simulink model "FlightDataRecorder"  (R2023b)
settings: Solver=VariableStepAuto  StartTime=0.0  StopTime=inf  RelTol=1e-3
libraries: dspindex x28, simulink x4, dspnetwork x4, etargetslib x3, aerolibconvert2 x1
(part 2 of 3)

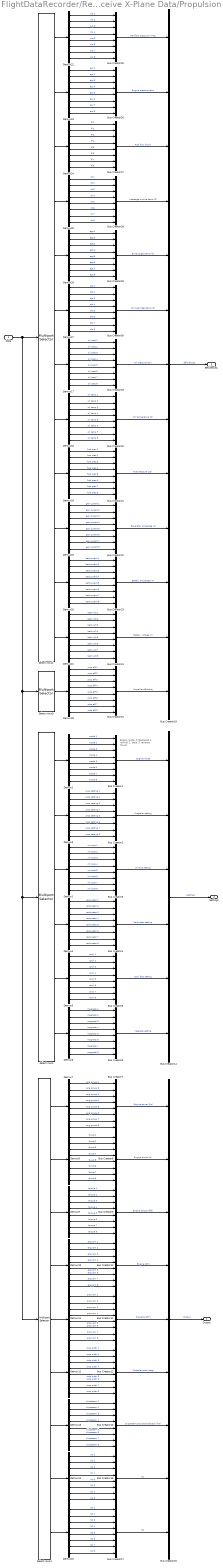
== system FlightDataRecorder/Receive X-Plane Data/Propulsion data ==
  note: Engine mode:
      | 0: feathered
      | 1: normal
      | 2: 'beta'
      | 3: reverse thrust
  Data : Inport
  Bus Creator{1..13,16..18,20..31} (28 alike) : BusCreator  Inputs=8
  Bus Creator14 : BusCreator  Inputs=6
  Bus Creator15 : BusCreator  Inputs=9
  Bus Creator19 : BusCreator  Inputs=13
  Demux{1..28} (28 alike) : Demux  Outputs=8
  Select rows : dspindex/Multiport Selector  rowsOrCols=Rows  idxCellArray={28,29,30,31,32,33}  idxErrMode=Clip Index
  Select rows1 : dspindex/Multiport Selector  rowsOrCols=Rows  idxCellArray={35,36,37,38,39,40,41,42,43}  idxErrMode=Clip Index
  Select rows2 : dspindex/Multiport Selector  rowsOrCols=Rows  idxCellArray={44,45,46,47,48,49,50,51,52,53,54,55}  idxErrMode=Clip Index
  Select rows3 : dspindex/Multiport Selector  rowsOrCols=Rows  idxCellArray={70}  idxErrMode=Clip Index
  Output : Outport
  Settings : Outport  Port=2
  Efficiencies : Outport  Port=3
  wires:
  Demux3/3 -> Bus Creator2/3  "prop setting 3"
  Demux3/2 -> Bus Creator2/2  "prop setting 2"
  Demux3/1 -> Bus Creator2/1  "prop setting 1"
  Demux3/4 -> Bus Creator2/4  "prop setting 4"
  Demux3/5 -> Bus Creator2/5  "prop setting 5"
  Demux3/6 -> Bus Creator2/6  "prop setting 6"
  Demux3/7 -> Bus Creator2/7  "prop setting 7"
  Demux3/8 -> Bus Creator2/8  "prop setting 8"
  Select rows/1 -> Demux2/1
  Select rows/2 -> Demux3/1
  Demux2/8 -> Bus Creator1/8  "mode 8"
  Demux2/1 -> Bus Creator1/1  "mode 1"
  Demux2/4 -> Bus Creator1/4  "mode 4"
  Demux2/7 -> Bus Creator1/7  "mode 7"
  Demux2/3 -> Bus Creator1/3  "mode 3"
  Demux2/5 -> Bus Creator1/5  "mode 5"
  Demux2/6 -> Bus Creator1/6  "mode 6"
  Demux2/2 -> Bus Creator1/2  "mode 2"
  Bus Creator1/1 -> Bus Creator14/1  "Engine mode"
  Bus Creator2/1 -> Bus Creator14/2  "Propeller setting"
  Demux1/3 -> Bus Creator3/3  "mixture 3"
  Demux1/4 -> Bus Creator3/4  "mixture 4"
  Demux1/5 -> Bus Creator3/5  "mixture 5"
  Demux1/6 -> Bus Creator3/6  "mixture 6"
  Demux1/7 -> Bus Creator3/7  "mixture 7"
  Demux1/8 -> Bus Creator3/8  "mixture 8"
  Select rows/3 -> Demux1/1
  Bus Creator3/1 -> Bus Creator14/3  "Mixture setting"
  Demux1/1 -> Bus Creator3/1  "mixture 1"
  Demux1/2 -> Bus Creator3/2  "mixture 2"
  Select rows/4 -> Demux4/1
  Demux4/4 -> Bus Creator4/4  "carburetor 4"
  Demux4/1 -> Bus Creator4/1  "carburetor 1"
  Demux4/6 -> Bus Creator4/6  "carburetor 6"
  Demux4/7 -> Bus Creator4/7  "carburetor 7"
  Demux4/5 -> Bus Creator4/5  "carburetor 5"
  Demux4/3 -> Bus Creator4/3  "carburetor 3"
  Demux4/2 -> Bus Creator4/2  "carburetor 2"
  Demux4/8 -> Bus Creator4/8  "carburetor 8"
  Bus Creator4/1 -> Bus Creator14/4  "Carburetor setting"
  Demux5/4 -> Bus Creator5/4  "cowl 4"
  Demux5/1 -> Bus Creator5/1  "cowl 1"
  Demux5/6 -> Bus Creator5/6  "cowl 6"
  Demux5/7 -> Bus Creator5/7  "cowl 7"
  Demux5/5 -> Bus Creator5/5  "cowl 5"
  Demux5/3 -> Bus Creator5/3  "cowl 3"
  Demux5/2 -> Bus Creator5/2  "cowl 2"
  Demux5/8 -> Bus Creator5/8  "cowl 8"
  Bus Creator5/1 -> Bus Creator14/5  "Cowl flap setting"
  Select rows/5 -> Demux5/1
  Demux6/4 -> Bus Creator6/4  "magneto 4"
  Demux6/1 -> Bus Creator6/1  "magneto 1"
  Demux6/6 -> Bus Creator6/6  "magneto 6"
  Demux6/7 -> Bus Creator6/7  "magneto 7"
  Demux6/5 -> Bus Creator6/5  "magneto 5"
  Demux6/3 -> Bus Creator6/3  "magneto 3"
  Demux6/2 -> Bus Creator6/2  "magneto 2"
  Demux6/8 -> Bus Creator6/8  "magneto 8"
  Bus Creator6/1 -> Bus Creator14/6  "Magneto setting"
  Select rows/6 -> Demux6/1
  Demux7/4 -> Bus Creator7/4  "eng power 4"
  Demux7/1 -> Bus Creator7/1  "eng power 1"
  Demux7/6 -> Bus Creator7/6  "eng power 6"
  Demux7/7 -> Bus Creator7/7  "eng power 7"
  Demux7/5 -> Bus Creator7/5  "eng power 5"
  Demux7/3 -> Bus Creator7/3  "eng power 3"
  Demux7/2 -> Bus Creator7/2  "eng power 2"
  Demux7/8 -> Bus Creator7/8  "eng power 8"
  Select rows1/1 -> Demux7/1
  Demux8/4 -> Bus Creator8/4  "thrust 4"
  Demux8/1 -> Bus Creator8/1  "thrust 1"
  Demux8/6 -> Bus Creator8/6  "thrust 6"
  Demux8/7 -> Bus Creator8/7  "thrust 7"
  Demux8/5 -> Bus Creator8/5  "thrust 5"
  Demux8/3 -> Bus Creator8/3  "thrust 3"
  Demux8/2 -> Bus Creator8/2  "thrust 2"
  Demux8/8 -> Bus Creator8/8  "thrust 8"
  Select rows1/2 -> Demux8/1
  Demux9/4 -> Bus Creator9/4  "torque 4"
  Demux9/1 -> Bus Creator9/1  "torque 1"
  Demux9/6 -> Bus Creator9/6  "torque 6"
  Demux9/7 -> Bus Creator9/7  "torque 7"
  Demux9/5 -> Bus Creator9/5  "torque 5"
  Demux9/3 -> Bus Creator9/3  "torque 3"
  Demux9/2 -> Bus Creator9/2  "torque 2"
  Demux9/8 -> Bus Creator9/8  "torque 8"
  Select rows1/3 -> Demux9/1
  Demux10/4 -> Bus Creator10/4  "eng rpm 4"
  Demux10/1 -> Bus Creator10/1  "eng rpm 1"
  Demux10/6 -> Bus Creator10/6  "eng rpm 6"
  Demux10/7 -> Bus Creator10/7  "eng rpm 7"
  Demux10/5 -> Bus Creator10/5  "eng rpm 5"
  Demux10/3 -> Bus Creator10/3  "eng rpm 3"
  Demux10/2 -> Bus Creator10/2  "eng rpm 2"
  Demux10/8 -> Bus Creator10/8  "eng rpm 8"
  Select rows1/4 -> Demux10/1
  Demux11/4 -> Bus Creator11/4  "prop rpm 4"
  Demux11/1 -> Bus Creator11/1  "prop rpm 1"
  Demux11/6 -> Bus Creator11/6  "prop rpm 6"
  Demux11/7 -> Bus Creator11/7  "prop rpm 7"
  Demux11/5 -> Bus Creator11/5  "prop rpm 5"
  Demux11/3 -> Bus Creator11/3  "prop rpm 3"
  Demux11/2 -> Bus Creator11/2  "prop rpm 2"
  Demux11/8 -> Bus Creator11/8  "prop rpm 8"
  Select rows1/5 -> Demux11/1
  Demux12/4 -> Bus Creator12/4  "prop pitch 4"
  Demux12/1 -> Bus Creator12/1  "prop pitch 1"
  Demux12/6 -> Bus Creator12/6  "prop pitch 6"
  Demux12/7 -> Bus Creator12/7  "prop pitch 7"
  Demux12/5 -> Bus Creator12/5  "prop pitch 5"
  Demux12/3 -> Bus Creator12/3  "prop pitch 3"
  Demux12/2 -> Bus Creator12/2  "prop pitch 2"
  Demux12/8 -> Bus Creator12/8  "prop pitch 8"
  Select rows1/6 -> Demux12/1
  Demux13/4 -> Bus Creator13/4  "slipstream 4"
  Demux13/1 -> Bus Creator13/1  "slipstream 1"
  Demux13/6 -> Bus Creator13/6  "slipstream 6"
  Demux13/7 -> Bus Creator13/7  "slipstream 7"
  Demux13/5 -> Bus Creator13/5  "slipstream 5"
  Demux13/3 -> Bus Creator13/3  "slipstream 3"
  Demux13/2 -> Bus Creator13/2  "slipstream 2"
  Demux13/8 -> Bus Creator13/8  "slipstream 8"
  Select rows1/7 -> Demux13/1
  Bus Creator14/1 -> Settings/1  "Settings"
  Bus Creator7/1 -> Bus Creator15/1  "Engine power (hp)"
  Bus Creator8/1 -> Bus Creator15/2  "Engine thrust (lb)"
  Bus Creator9/1 -> Bus Creator15/3  "Engine torque (ftlb)"
  Bus Creator10/1 -> Bus Creator15/4  "Engine RPM"
  Bus Creator11/1 -> Bus Creator15/5  "Propeller RPM"
  Bus Creator12/1 -> Bus Creator15/6  "Propeller pitch (deg)"
  Bus Creator13/1 -> Bus Creator15/7  "Slipstream/propwash/jetwash (knt)"
  Bus Creator15/1 -> Output/1  "Output"
  Demux14/4 -> Bus Creator16/4  "N1 4"
  Demux14/6 -> Bus Creator16/6  "N1 6"
  Demux14/7 -> Bus Creator16/7  "N1 7"
  Demux14/5 -> Bus Creator16/5  "N1 5"
  Demux14/3 -> Bus Creator16/3  "N1 3"
  Demux14/2 -> Bus Creator16/2  "N1 2"
  Demux14/8 -> Bus Creator16/8  "N1 8"
  Select rows1/8 -> Demux14/1
  Demux15/4 -> Bus Creator17/4  "N2 4"
  Demux15/6 -> Bus Creator17/6  "N2 6"
  Demux15/7 -> Bus Creator17/7  "N2 7"
  Demux15/5 -> Bus Creator17/5  "N2 5"
  Demux15/3 -> Bus Creator17/3  "N2 3"
  Demux15/2 -> Bus Creator17/2  "N2 2"
  Demux15/8 -> Bus Creator17/8  "N2 8"
  Select rows1/9 -> Demux15/1
  Demux14/1 -> Bus Creator16/1  "N1 1"
  Demux15/1 -> Bus Creator17/1  "N2 1"
  Bus Creator16/1 -> Bus Creator15/8  "N1"
  Bus Creator17/1 -> Bus Creator15/9  "N2"
  Demux18/3 -> Bus Creator20/3  "oil temp 3"
  Demux18/2 -> Bus Creator20/2  "oil temp 2"
  Demux18/1 -> Bus Creator20/1  "oil temp 1"
  Data/1 -> Select rows3/1, Select rows/1, Select rows1/1, Select rows2/1
  Demux18/4 -> Bus Creator20/4  "oil temp 4"
  Demux18/5 -> Bus Creator20/5  "oil temp 5"
  Demux18/6 -> Bus Creator20/6  "oil temp 6"
  Demux18/7 -> Bus Creator20/7  "oil temp 7"
  Demux18/8 -> Bus Creator20/8  "oil temp 8"
  Demux17/8 -> Bus Creator18/8  "oil pres 8"
  Demux17/1 -> Bus Creator18/1  "oil pres 1"
  Demux17/4 -> Bus Creator18/4  "oil pres 4"
  Demux17/7 -> Bus Creator18/7  "oil pres 7"
  Demux17/3 -> Bus Creator18/3  "oil pres 3"
  Demux17/5 -> Bus Creator18/5  "oil pres 5"
  Demux17/6 -> Bus Creator18/6  "oil pres 6"
  Demux17/2 -> Bus Creator18/2  "oil pres 2"
  Demux16/3 -> Bus Creator21/3  "fuel pres 3"
  Demux16/4 -> Bus Creator21/4  "fuel pres 4"
  Demux16/5 -> Bus Creator21/5  "fuel pres 5"
  Demux16/6 -> Bus Creator21/6  "fuel pres 6"
  Demux16/7 -> Bus Creator21/7  "fuel pres 7"
  Demux16/8 -> Bus Creator21/8  "fuel pres 8"
  Demux16/1 -> Bus Creator21/1  "fuel pres 1"
  Demux16/2 -> Bus Creator21/2  "fuel pres 2"
  Demux19/4 -> Bus Creator22/4  "gen current 4"
  Demux19/1 -> Bus Creator22/1  "gen current 1"
  Demux19/6 -> Bus Creator22/6  "gen current 6"
  Demux19/7 -> Bus Creator22/7  "gen current 7"
  Demux19/5 -> Bus Creator22/5  "gen current 5"
  Demux19/3 -> Bus Creator22/3  "gen current 3"
  Demux19/2 -> Bus Creator22/2  "gen current 2"
  Demux19/8 -> Bus Creator22/8  "gen current 8"
  Demux20/4 -> Bus Creator23/4  "batt current 4"
  Demux20/1 -> Bus Creator23/1  "batt current 1"
  Demux20/6 -> Bus Creator23/6  "batt current 6"
  Demux20/7 -> Bus Creator23/7  "batt current 7"
  Demux20/5 -> Bus Creator23/5  "batt current 5"
  Demux20/3 -> Bus Creator23/3  "batt current 3"
  Demux20/2 -> Bus Creator23/2  "batt current 2"
  Demux20/8 -> Bus Creator23/8  "batt current 8"
  Demux21/1 -> Bus Creator24/1  "batt volt 1"
  Demux21/2 -> Bus Creator24/2  "batt volt 2"
  Bus Creator19/1 -> Efficiencies/1  "Efficiencies"
  Select rows2/12 -> Demux21/1
  Select rows2/11 -> Demux20/1
  Select rows2/10 -> Demux19/1
  Select rows2/9 -> Demux16/1
  Select rows2/7 -> Demux17/1
  Select rows2/8 -> Demux18/1
  Demux21/7 -> Bus Creator24/7  "batt volt 7"
  Demux21/6 -> Bus Creator24/6  "batt volt 6"
  Demux21/8 -> Bus Creator24/8  "batt volt 8"
  Demux21/3 -> Bus Creator24/3  "batt volt 3"
  Demux21/5 -> Bus Creator24/5  "batt volt 5"
  Demux21/4 -> Bus Creator24/4  "batt volt 4"
  Bus Creator18/1 -> Bus Creator19/7  "Oil pressure (psi)"
  Bus Creator20/1 -> Bus Creator19/8  "Oil temperature (C)"
  Bus Creator21/1 -> Bus Creator19/9  "Fuel pressure (psi)"
  Bus Creator22/1 -> Bus Creator19/10  "Generator amperage (A)"
  Bus Creator23/1 -> Bus Creator19/11  "Battery amperage (A)"
  Bus Creator24/1 -> Bus Creator19/12  "Battery voltage (V)"
  Demux22/8 -> Bus Creator25/8  "mp 8"
  Demux22/1 -> Bus Creator25/1  "mp 1"
  Demux22/4 -> Bus Creator25/4  "mp 4"
  Demux22/7 -> Bus Creator25/7  "mp 7"
  Demux22/3 -> Bus Creator25/3  "mp 3"
  Demux22/5 -> Bus Creator25/5  "mp 5"
  Demux22/6 -> Bus Creator25/6  "mp 6"
  Demux22/2 -> Bus Creator25/2  "mp 2"
  Select rows2/1 -> Demux22/1
  Bus Creator25/1 -> Bus Creator19/1  "Manifold pressure (inHg)"
  Demux23/8 -> Bus Creator26/8  "epr 8"
  Demux23/7 -> Bus Creator26/7  "epr 7"
  Select rows2/2 -> Demux23/1
  Bus Creator26/1 -> Bus Creator19/2  "Engine pressure ratio"
  Demux23/6 -> Bus Creator26/6  "epr 6"
  Demux23/4 -> Bus Creator26/4  "epr 4"
  Demux23/1 -> Bus Creator26/1  "epr 1"
  Demux23/2 -> Bus Creator26/2  "epr 2"
  Demux23/3 -> Bus Creator26/3  "epr 3"
  Demux23/5 -> Bus Creator26/5  "epr 5"
  Demux24/8 -> Bus Creator27/8  "ff 8"
  Demux24/7 -> Bus Creator27/7  "ff 7"
  Demux24/6 -> Bus Creator27/6  "ff 6"
  Demux24/4 -> Bus Creator27/4  "ff 4"
  Demux24/1 -> Bus Creator27/1  "ff 1"
  Demux24/2 -> Bus Creator27/2  "ff 2"
  Demux24/3 -> Bus Creator27/3  "ff 3"
  Demux24/5 -> Bus Creator27/5  "ff 5"
  Select rows2/3 -> Demux24/1
  Bus Creator27/1 -> Bus Creator19/3  "Fuel flow (lb/hr)"
  Demux25/8 -> Bus Creator28/8  "itt 8"
  Demux25/7 -> Bus Creator28/7  "itt 7"
  Demux25/6 -> Bus Creator28/6  "itt 6"
  Demux25/4 -> Bus Creator28/4  "itt 4"
  Demux25/1 -> Bus Creator28/1  "itt 1"
  Demux25/2 -> Bus Creator28/2  "itt 2"
  Demux25/3 -> Bus Creator28/3  "itt 3"
  Demux25/5 -> Bus Creator28/5  "itt 5"
  Select rows2/4 -> Demux25/1
  Bus Creator28/1 -> Bus Creator19/4  "Interstage turbine temp (C)"
  Demux26/8 -> Bus Creator29/8  "egt 8"
  Demux26/7 -> Bus Creator29/7  "egt 7"
  Demux26/6 -> Bus Creator29/6  "egt 6"
  Demux26/4 -> Bus Creator29/4  "egt 4"
  Demux26/2 -> Bus Creator29/2  "egt 2"
  Demux26/3 -> Bus Creator29/3  "egt 3"
  Demux26/5 -> Bus Creator29/5  "egt 5"
  Select rows2/5 -> Demux26/1
  Bus Creator29/1 -> Bus Creator19/5  "Exhaust gas temp (C)"
  Demux27/8 -> Bus Creator30/8  "cht 8"
  Demux27/7 -> Bus Creator30/7  "cht 7"
  Demux27/6 -> Bus Creator30/6  "cht 6"
  Demux27/4 -> Bus Creator30/4  "cht 4"
  Demux27/2 -> Bus Creator30/2  "cht 2"
  Demux27/3 -> Bus Creator30/3  "cht 3"
  Demux27/5 -> Bus Creator30/5  "cht 5"
  Select rows2/6 -> Demux27/1
  Demux27/1 -> Bus Creator30/1  "cht 1"
  Bus Creator30/1 -> Bus Creator19/6  "Cylinder head temp (C)"
  Demux26/1 -> Bus Creator29/1  "egt 1"
  Demux28/8 -> Bus Creator31/8  "prop eff 8"
  Demux28/1 -> Bus Creator31/1  "prop eff 1"
  Demux28/4 -> Bus Creator31/4  "prop eff 4"
  Demux28/7 -> Bus Creator31/7  "prop eff 7"
  Demux28/3 -> Bus Creator31/3  "prop eff 3"
  Demux28/5 -> Bus Creator31/5  "prop eff 5"
  Demux28/6 -> Bus Creator31/6  "prop eff 6"
  Demux28/2 -> Bus Creator31/2  "prop eff 2"
  Select rows3/1 -> Demux28/1
  Bus Creator31/1 -> Bus Creator19/13  "Propeller efficiency"

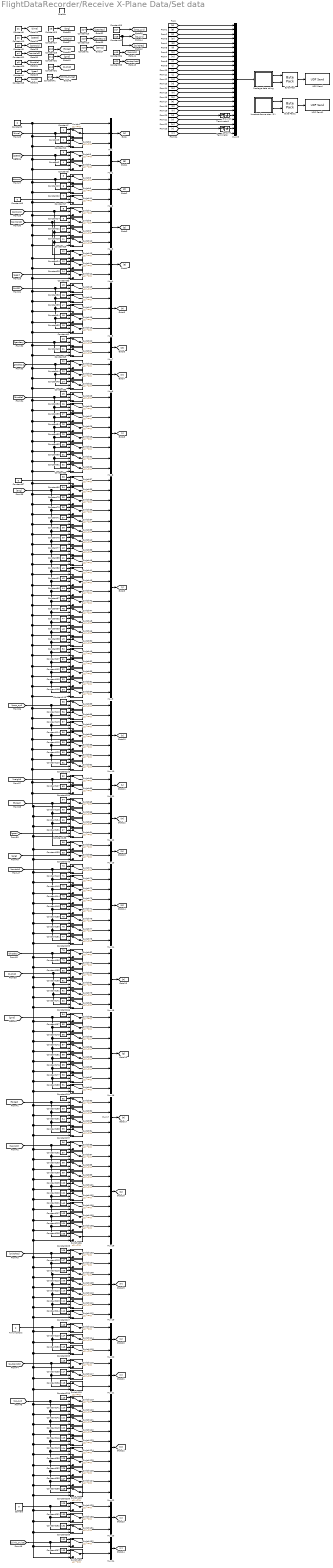
== system FlightDataRecorder/Receive X-Plane Data/Set data ==
  Enable : EnablePort
  Annunciators : Constant  Value=0
  Byte Pack : etargetslib/Byte Pack  datatypes={'uint8','uint32'}  byteAlign=1
  Byte Pack1 : etargetslib/Byte Pack  datatypes={'uint8','uint32'}  byteAlign=1
  Camera : Constant  Value=0
  Constant1 : Constant  Value=p16
  Constant10 : Constant  Value=p2
  Constant102 : Constant  Value=52
  Constant103 : Constant  Value=53
  Constant107 : Constant  Value=51
  Constant108 : Constant  Value=54
  Constant11 : Constant  Value=p4
  Constant110 : Constant  Value=56
  Constant113 : Constant  Value=55
  Constant114 : Constant  Value=58
  Constant115 : Constant  Value=59
  Constant119 : Constant  Value=57
  Constant12 : Constant  Value=3
  Constant120 : Constant  Value=61
  Constant125 : Constant  Value=60
  Constant126 : Constant  Value=62
  Constant127 : Constant  Value=63
  Constant128 : Constant  Value=65
  Constant13 : Constant  Value=6
  Constant131 : Constant  Value=67
  Constant134 : Constant  Value=66
  Constant135 : Constant  Value=64
  Constant138 : Constant  Value=68
  Constant139 : Constant  Value=69
  Constant14 : Constant  Value=9
  Constant140 : Constant  Value=71
  Constant143 : Constant  Value=70
  Constant144 : Constant  Value=73
  Constant145 : Constant  Value=74
  Constant149 : Constant  Value=72
  Constant15 : Constant  Value=p7
  Constant150 : Constant  Value=76
  Constant151 : Constant  Value=77
  Constant155 : Constant  Value=75
  Constant156 : Constant  Value=79
  Constant159 : Constant  Value=78
  Constant16 : Constant  Value=p14
  Constant160 : Constant  Value=81
  Constant161 : Constant  Value=82
  Constant165 : Constant  Value=80
  Constant166 : Constant  Value=84
  Constant167 : Constant  Value=85
  Constant17 : Constant  Value=8
  Constant171 : Constant  Value=83
  Constant172 : Constant  Value=87
  Constant175 : Constant  Value=86
  Constant176 : Constant  Value=89
  Constant177 : Constant  Value=90
  Constant18 : Constant  Value=11
  Constant181 : Constant  Value=88
  Constant183 : Constant  Value=91
  Constant184 : Constant  Value=92
  Constant185 : Constant  Value=93
  Constant188 : Constant  Value=95
  Constant19 : Constant  Value=p15
  Constant191 : Constant  Value=94
  Constant192 : Constant  Value=97
  Constant193 : Constant  Value=98
  Constant197 : Constant  Value=96
  Constant199 : Constant  Value=99
  Constant2 : Constant  Value=4
  Constant20 : Constant  Value=p5
  Constant200 : Constant  Value=101
  Constant201 : Constant  Value=102
  Constant205 : Constant  Value=100
  Constant207 : Constant  Value=103
  Constant208 : Constant  Value=105
  Constant209 : Constant  Value=106
  Constant21 : Constant  Value=10
  Constant213 : Constant  Value=104
  Constant215 : Constant  Value=107
  Constant216 : Constant  Value=108
  Constant219 : Constant  Value=109
  Constant22 : Constant  Value=7
  Constant220 : Constant  Value=110
  Constant223 : Constant  Value=111
  Constant224 : Constant  Value=112
  Constant227 : Constant  Value=113
  Constant229 : Constant  Value=114
  Constant23 : Constant  Value=p8
  Constant230 : Constant  Value=115
  Constant233 : Constant  Value=116
  Constant235 : Constant  Value=117
  Constant236 : Constant  Value=118
  Constant238 : Constant  Value=119
  Constant24 : Constant  Value=13
  Constant241 : Constant  Value=120
  Constant242 : Constant  Value=121
  Constant245 : Constant  Value=122
  Constant246 : Constant  Value=123
  Constant249 : Constant  Value=124
  Constant25 : Constant  Value=14
  Constant250 : Constant  Value=125
  Constant252 : Constant  Value=126
  Constant255 : Constant  Value=127
  Constant256 : Constant  Value=128
  Constant259 : Constant  Value=129
  Constant26 : Constant  Value=p17
  Constant261 : Constant  Value=130
  Constant262 : Constant  Value=131
  Constant265 : Constant  Value=132
  Constant267 : Constant  Value=133
  Constant27 : Constant  Value=p9
  Constant28 : Constant  Value=p10
  Constant29 : Constant  Value=12
  Constant3 : Constant  Value=p3
  Constant30 : Constant  Value=16
  Constant31 : Constant  Value=p12
  Constant32 : Constant  Value=p11
  Constant33 : Constant  Value=15
  Constant34 : Constant  Value=18
  Constant35 : Constant  Value=19
  Constant36 : Constant  Value=p19
  Constant37 : Constant  Value=0
  Constant38 : Constant  Value=p20
  Constant39 : Constant  Value=17
  Constant4 : Constant  Value=p6
  Constant40 : Constant  Value=p18
  Constant41 : Constant  Value=p13
  Constant42 : Constant  Value=20
  Constant43 : Constant  Value=21
  Constant44 : Constant  Value=23
  Constant45 : Constant  Value=24
  Constant46 : Constant  Value=0
  Constant49 : Constant  Value=22
  Constant5 : Constant  Value=0
  Constant50 : Constant  Value=26
  Constant53 : Constant  Value=25
  Constant54 : Constant  Value=28
  Constant55 : Constant  Value=29
  Constant59 : Constant  Value=27
  Constant6 : Constant  Value=5
  Constant60 : Constant  Value=31
  Constant61 : Constant  Value=32
  Constant65 : Constant  Value=30
  Constant66 : Constant  Value=34
  Constant69 : Constant  Value=33
  Constant7 : Constant
  Constant70 : Constant  Value=36
  Constant71 : Constant  Value=37
  Constant75 : Constant  Value=35
  Constant76 : Constant  Value=39
  Constant77 : Constant  Value=40
  Constant8 : Constant  Value=p1
  Constant81 : Constant  Value=38
  Constant82 : Constant  Value=42
  Constant85 : Constant  Value=41
  Constant86 : Constant  Value=44
  Constant87 : Constant  Value=45
  Constant9 : Constant  Value=2
  Constant91 : Constant  Value=43
  Constant92 : Constant  Value=47
  Constant93 : Constant  Value=48
  Constant97 : Constant  Value=46
  Constant98 : Constant  Value=49
  Constant99 : Constant  Value=50
  From : From
  Goto : Goto
  Ground : Ground
  Ground1 : Ground
  Mux{,2,4,6,20..21,23} (7 alike) : Mux  Inputs=3
  Mux{1,7,11,13,24} (5 alike) : Mux  Inputs=2
  Mux10 : Mux  Inputs=7
  Mux12 : Mux
  Mux14 : Mux  Inputs=8
  Mux15 : Mux  Inputs=6
  Mux16 : Mux  Inputs=8
  Mux17 : Mux
  Mux18 : Mux  Inputs=10
  Mux19 : Mux  Inputs=7
  Mux22 : Mux  Inputs=10
  Mux25 : Mux  Inputs=25
  Mux3 : Mux
  Mux5 : Mux  Inputs=5
  Mux8 : Mux  Inputs=8
  Mux9 : Mux  Inputs=22
  Package data string : MATLAB Function  TreatAsAtomicUnit=on
  Switch{1..133} (133 alike) : Switch  Criteria=u2 ~= 0  SaturateOnIntegerOverflow=off  InputSameDT=off
  Terminator : Terminator
  Terminator1 : Terminator
  UDP Send : dspnetwork/UDP Send  remoteURL=ipaddress  remotePort=sport  localURL='0.0.0.0'  localPortSource=Automatically determine  localPort=-1  sendBufferSize=8192  sampletime=-1  blockPlatform=[]  separateLengthPort=0
  UDP Send1 : dspnetwork/UDP Send  remoteURL=ipaddress  remotePort=sport  localURL='0.0.0.0'  localPortSource=Automatically determine  localPort=-1  sendBufferSize=8192  sampletime=-1  blockPlatform=[]  separateLengthPort=0
  Unselect frame rate <0> : MATLAB Function  TreatAsAtomicUnit=on
  wires:
  Constant7/1 -> Switch1/1
  [time] -> Switch2/2, Switch1/2
  Constant9/1 -> Switch2/1
  Constant12/1 -> Switch3/1
  [speed] -> Switch4/2, Switch3/2
  Constant2/1 -> Switch4/1
  Switch1/1 -> Mux/2
  Switch2/1 -> Mux/3
  Switch3/1 -> Mux1/1
  Switch4/1 -> Mux1/2
  Constant6/1 -> Switch5/1
  [atmos] -> Switch6/2, Switch5/2
  Constant13/1 -> Switch6/1
  Constant17/1 -> Switch7/1
  [controls] -> Switch7/2, Switch14/2, Switch10/2, Switch9/2
  Constant14/1 -> Switch8/1
  Constant21/1 -> Switch9/1
  Constant18/1 -> Switch10/1
  Switch7/1 -> Mux3/1
  Switch8/1 -> Mux3/2
  Switch9/1 -> Mux3/3
  Switch10/1 -> Mux3/4
  Switch5/1 -> Mux2/1
  Switch6/1 -> Mux2/2
  Constant22/1 -> Switch11/1
  Switch11/1 -> Mux2/3
  Constant29/1 -> Switch13/1
  Constant24/1 -> Switch14/1
  Switch13/1 -> Mux4/1
  Switch14/1 -> Mux4/2
  Constant25/1 -> Switch12/1
  [gear] -> Switch12/2
  Switch12/1 -> Mux4/3
  Constant33/1 -> Switch19/1
  [AHRS] -> Switch16/2, Switch18/2, Switch17/2, Switch15/2, Switch19/2
  Constant30/1 -> Switch15/1
  Constant39/1 -> Switch17/1
  Constant34/1 -> Switch18/1
  Constant35/1 -> Switch16/1
  Switch18/1 -> Mux5/4
  Switch15/1 -> Mux5/2
  Switch16/1 -> Mux5/5
  Switch17/1 -> Mux5/3
  Switch19/1 -> Mux5/1
  Constant42/1 -> Switch20/1
  [geodesy] -> Switch21/2, Switch20/2
  Constant43/1 -> Switch21/1
  Switch20/1 -> Mux7/1
  Switch21/1 -> Mux7/2
  Constant5/1 -> Mux/1, Switch5/3, Switch11/3, Switch7/3, Switch8/3, Switch9/3, Switch13/3, Switch14/3, Switch12/3, Switch19/3, Switch15/3, Switch17/3, Switch18/3, Switch16/3, Switch20/3, Switch23/3, Switch24/3, Switch22/3, Switch29/3, Switch25/3, Switch27/3, Switch28/3, Switch26/3, Switch31/3, Switch32/3, Switch37/3, Switch33/3, Switch35/3, Switch36/3, Switch34/3, Switch39/3, Switch40/3, Switch38/3, Switch45/3, Switch41/3, Switch43/3, Switch44/3, Switch42/3, Switch47/3, Switch48/3, Switch46/3, Switch50/3, Switch49/3, Switch52/3, Switch53/3, Switch51/3, Switch59/3, Switch55/3, Switch57/3, Switch58/3, Switch56/3, Switch61/3, Switch66/3, Switch67/3, Switch74/3, Switch70/3, Switch72/3, Switch73/3, Switch71/3, Switch76/3, Switch77/3, Switch82/3, Switch78/3, Switch80/3, Switch81/3, Switch79/3, Switch84/3, Switch85/3, Switch90/3, Switch86/3, Switch88/3, Switch89/3, Switch87/3, Switch93/3, Switch92/3, Switch98/3, Switch97/3, Switch95/3, Switch99/3, Switch101/3, Switch102/3, Switch100/3, Switch103/3, Switch105/3, Switch104/3, Switch107/3, Switch108/3, Switch109/3, Switch110/3, Switch111/3, Switch113/3, Switch114/3, Switch115/3, Switch116/3, Switch117/3, Switch119/3, Switch120/3, Switch121/3, Switch122/3, Switch123/3, Switch124/3, Switch125/3, Switch126/3, Switch127/3, Switch129/3, Switch130/3, Switch131/3, Switch132/3, Switch133/3, Switch128/3, Switch118/3, Switch112/3, Switch106/3, Switch96/3, Switch94/3, Switch91/3, Switch83/3, Switch75/3, Switch69/3, Switch68/3, Switch64/3, Switch65/3, Switch63/3, Switch60/3, Switch62/3, Switch54/3, Switch30/3, Switch21/3, Switch10/3, Switch6/3, Switch4/3, Switch3/3, Switch2/3, Switch1/3
  Constant49/1 -> Switch23/1
  [geodesy2] -> Switch22/2, Switch24/2, Switch23/2
  Constant44/1 -> Switch24/1
  Switch23/1 -> Mux6/1
  Switch24/1 -> Mux6/2
  Constant45/1 -> Switch22/1
  Switch22/1 -> Mux6/3
  Constant53/1 -> Switch29/1
  [throttle] -> Switch30/2, Switch32/2, Switch31/2, Switch26/2, Switch28/2, Switch27/2, Switch25/2, Switch29/2
  Constant50/1 -> Switch25/1
  Constant59/1 -> Switch27/1
  Constant54/1 -> Switch28/1
  Constant55/1 -> Switch26/1
  Switch28/1 -> Mux8/4
  Switch25/1 -> Mux8/2
  Switch26/1 -> Mux8/5
  Switch27/1 -> Mux8/3
  Switch29/1 -> Mux8/1
  Constant60/1 -> Switch32/1
  Constant61/1 -> Switch30/1
  Switch32/1 -> Mux8/7
  Switch30/1 -> Mux8/8
  Switch31/1 -> Mux8/6
  Constant69/1 -> Switch37/1
  Constant66/1 -> Switch33/1
  [eng] -> Switch54/2, Switch51/2, Switch53/2, Switch52/2, Switch49/2, Switch50/2, Switch46/2, Switch48/2, Switch47/2, Switch42/2, Switch44/2, Switch43/2, Switch41/2, Switch45/2, Switch38/2, Switch40/2, Switch39/2, Switch34/2, Switch36/2, Switch35/2, Switch33/2
  Constant75/1 -> Switch35/1
  Constant70/1 -> Switch36/1
  Constant71/1 -> Switch34/1
  Switch36/1 -> Mux9/4
  Switch33/1 -> Mux9/2
  Switch34/1 -> Mux9/5
  Switch35/1 -> Mux9/3
  Switch37/1 -> Mux9/1
  Constant76/1 -> Switch40/1
  Constant77/1 -> Switch38/1
  Switch40/1 -> Mux9/7
  Switch38/1 -> Mux9/8
  Switch39/1 -> Mux9/6
  Constant85/1 -> Switch45/1
  Constant82/1 -> Switch41/1
  Constant91/1 -> Switch43/1
  Constant86/1 -> Switch44/1
  Constant87/1 -> Switch42/1
  Switch44/1 -> Mux9/12
  Switch41/1 -> Mux9/10
  Switch42/1 -> Mux9/13
  Switch43/1 -> Mux9/11
  Switch45/1 -> Mux9/9
  Constant92/1 -> Switch48/1
  Constant93/1 -> Switch46/1
  Switch48/1 -> Mux9/15
  Switch46/1 -> Mux9/16
  Switch47/1 -> Mux9/14
  Constant98/1 -> Switch50/1
  Constant99/1 -> Switch49/1
  Switch50/1 -> Mux9/17
  Switch49/1 -> Mux9/18
  Constant102/1 -> Switch53/1
  Constant103/1 -> Switch51/1
  Switch53/1 -> Mux9/20
  Switch51/1 -> Mux9/21
  Switch52/1 -> Mux9/19
  Constant108/1 -> Switch54/1
  Switch54/1 -> Mux9/22
  Constant113/1 -> Switch59/1
  Constant110/1 -> Switch55/1
  Constant119/1 -> Switch57/1
  Constant114/1 -> Switch58/1
  Constant115/1 -> Switch56/1
  Switch58/1 -> Mux10/4
  Switch55/1 -> Mux10/2
  Switch56/1 -> Mux10/5
  Switch57/1 -> Mux10/3
  Switch59/1 -> Mux10/1
  Constant120/1 -> Switch62/1
  [prop_sys] -> Switch55/2, Switch57/2, Switch58/2, Switch56/2, Switch61/2, Switch62/2, Switch59/2
  Switch62/1 -> Mux10/7
  Switch61/1 -> Mux10/6
  Constant126/1 -> Switch60/1
  Constant127/1 -> Switch63/1
  [weight] -> Switch63/2, Switch60/2
  Switch60/1 -> Mux11/1
  Switch63/1 -> Mux11/2
  Constant128/1 -> Switch66/1
  Constant134/1 -> Switch67/1
  Constant131/1 -> Switch64/1
  [forces] -> Switch68/2, Switch67/2, Switch66/2, Switch65/2
  Switch65/1 -> Mux12/1
  Switch66/1 -> Mux12/2
  Switch67/1 -> Mux12/3
  Switch64/1 -> Mux12/4
  Constant135/1 -> Switch65/1
  Constant138/1 -> Switch68/1
  Constant139/1 -> Switch69/1
  Switch68/1 -> Mux13/1
  Switch69/1 -> Mux13/2
  Constant143/1 -> Switch74/1
  Constant140/1 -> Switch70/1
  Constant149/1 -> Switch72/1
  Constant144/1 -> Switch73/1
  Constant145/1 -> Switch71/1
  Switch73/1 -> Mux14/4
  Switch70/1 -> Mux14/2
  Switch71/1 -> Mux14/5
  Switch72/1 -> Mux14/3
  Switch74/1 -> Mux14/1
  Constant150/1 -> Switch77/1
  Constant151/1 -> Switch75/1
  [controls] -> Switch70/2, Switch72/2, Switch73/2, Switch71/2, Switch76/2, Switch77/2, Switch75/2, Switch74/2
  Switch77/1 -> Mux14/7
  Switch75/1 -> Mux14/8
  Switch76/1 -> Mux14/6
  Constant159/1 -> Switch82/1
  [throttle] -> Switch78/2, Switch82/2
  Constant156/1 -> Switch78/1
  Constant165/1 -> Switch80/1
  Constant160/1 -> Switch81/1
  Constant161/1 -> Switch79/1
  Switch81/1 -> Mux15/4
  Switch78/1 -> Mux15/2
  Switch79/1 -> Mux15/5
  Switch80/1 -> Mux15/3
  Switch82/1 -> Mux15/1
  Constant166/1 -> Switch85/1
  Constant167/1 -> Switch83/1
  Switch84/1 -> Mux15/6
  Switch85/1 -> Mux16/1
  Switch83/1 -> Mux16/2
  Constant175/1 -> Switch90/1
  Constant172/1 -> Switch86/1
  Constant181/1 -> Switch88/1
  Constant176/1 -> Switch89/1
  Constant177/1 -> Switch87/1
  Switch89/1 -> Mux16/6
  Switch86/1 -> Mux16/4
  Switch87/1 -> Mux16/7
  Switch88/1 -> Mux16/5
  Switch90/1 -> Mux16/3
  [grnd] -> Switch83/2, Switch90/2, Switch86/2, Switch88/2, Switch89/2, Switch87/2, Switch91/2, Switch85/2
  Switch91/1 -> Mux16/8
  Constant184/1 -> Switch93/1
  Constant185/1 -> Switch92/1
  Switch93/1 -> Mux17/1
  Switch92/1 -> Mux17/2
  Constant191/1 -> Switch98/1
  Constant188/1 -> Switch94/1
  [forces] -> Switch92/2, Switch98/2, Switch94/2, Switch93/2
  Constant197/1 -> Switch96/1
  [NAVAID] -> Switch97/2, Switch95/2, Switch99/2, Switch101/2, Switch102/2, Switch100/2, Switch103/2, Switch105/2, Switch106/2, Switch96/2
  Constant192/1 -> Switch97/1
  Constant193/1 -> Switch95/1
  Switch94/1 -> Mux17/4
  Switch98/1 -> Mux17/3
  Switch96/1 -> Mux18/1
  Switch97/1 -> Mux18/2
  Switch95/1 -> Mux18/3
  Switch99/1 -> Mux18/4
  Constant205/1 -> Switch101/1
  Constant200/1 -> Switch102/1
  Constant201/1 -> Switch100/1
  Switch101/1 -> Mux18/5
  Switch102/1 -> Mux18/6
  Switch100/1 -> Mux18/7
  Switch103/1 -> Mux18/8
  Constant213/1 -> Switch105/1
  Constant208/1 -> Switch106/1
  Constant209/1 -> Switch104/1
  [switches] -> Switch112/2, Switch111/2, Switch110/2, Switch109/2, Switch108/2, Switch107/2, Switch104/2
  Switch105/1 -> Mux18/9
  Switch106/1 -> Mux18/10
  Switch104/1 -> Mux19/1
  Switch107/1 -> Mux19/2
  Constant216/1 -> Switch108/1
  Constant220/1 -> Switch110/1
  Constant224/1 -> Switch112/1
  Switch108/1 -> Mux19/3
  Switch109/1 -> Mux19/4
  Switch110/1 -> Mux19/5
  Switch111/1 -> Mux19/6
  Switch112/1 -> Mux19/7
  Constant207/1 -> Switch103/1
  Constant155/1 -> Switch76/1
  Constant107/1 -> Switch52/1
  Constant81/1 -> Switch39/1
  Constant65/1 -> Switch31/1
  Constant97/1 -> Switch47/1
  Constant125/1 -> Switch61/1
  Constant183/1 -> Switch91/1
  Constant215/1 -> Switch107/1
  Constant227/1 -> Switch113/1
  Annunciators/1 -> Switch115/2, Switch114/2, Switch113/2
  Constant230/1 -> Switch115/1
  Switch114/1 -> Mux20/2
  Switch115/1 -> Mux20/3
  Constant223/1 -> Switch111/1
  Constant219/1 -> Switch109/1
  Switch113/1 -> Mux20/1
  Constant229/1 -> Switch114/1
  Constant233/1 -> Switch116/1
  Constant236/1 -> Switch118/1
  [autopilots] -> Switch117/2, Switch118/2, Switch116/2
  Switch117/1 -> Mux21/2
  Switch118/1 -> Mux21/3
  Switch116/1 -> Mux21/1
  Constant235/1 -> Switch117/1
  Constant238/1 -> Switch119/1
  Constant242/1 -> Switch121/1
  Constant246/1 -> Switch123/1
  Constant250/1 -> Switch125/1
  Constant241/1 -> Switch120/1
  Constant249/1 -> Switch124/1
  Constant245/1 -> Switch122/1
  Switch119/1 -> Mux22/1
  Switch120/1 -> Mux22/2
  Switch121/1 -> Mux22/3
  Switch122/1 -> Mux22/4
  Switch123/1 -> Mux22/5
  Switch124/1 -> Mux22/6
  Switch125/1 -> Mux22/7
  Constant252/1 -> Switch126/1
  Constant256/1 -> Switch128/1
  Constant255/1 -> Switch127/1
  Switch126/1 -> Mux22/8
  Switch127/1 -> Mux22/9
  Switch128/1 -> Mux22/10
  Constant262/1 -> Switch131/1
  Switch130/1 -> Mux23/2
  Switch131/1 -> Mux23/3
  Switch129/1 -> Mux23/1
  Constant261/1 -> Switch130/1
  [climb_cruise] -> Switch133/2, Switch132/2
  Switch133/1 -> Mux24/2
  Switch132/1 -> Mux24/1
  Constant267/1 -> Switch133/1
  Constant259/1 -> Switch129/1
  Constant265/1 -> Switch132/1
  Constant171/1 -> Switch84/1
  Constant199/1 -> Switch99/1
  Mux/1 -> Goto/1
  Mux1/1 -> [B]
  Mux2/1 -> [C]
  Mux5/1 -> [F]
  Mux7/1 -> [G]
  Mux6/1 -> [H]
  Mux8/1 -> [I]
  Mux3/1 -> [D]
  Mux4/1 -> [E]
  Mux9/1 -> [J]
  Mux10/1 -> [K]
  Mux11/1 -> [L]
  Mux12/1 -> [M]
  Mux13/1 -> [N]
  Mux14/1 -> [O]
  Mux15/1 -> [P]
  Mux16/1 -> [Q]
  Mux17/1 -> [R]
  Mux18/1 -> [S]
  Mux19/1 -> [T]
  Mux20/1 -> [U]
  Mux21/1 -> [V]
  Mux22/1 -> [W]
  Mux23/1 -> [X]
  Mux24/1 -> [Y]
  From/1 -> Mux25/1  "time"
  Mux25/1 -> Package data string/1(u)
  [B] -> Mux25/2  "speeds"
  [C] -> Mux25/3  "atmospherics"
  [D] -> Mux25/4  "flight controls"
  [E] -> Mux25/5  "landing gear"
  [G] -> Mux25/7  "geodesy"
  [M] -> Mux25/13  "forces"
  [L] -> Mux25/12  "weights"
  [K] -> Mux25/11  "propulsion systems"
  [J] -> Mux25/10  "engine thrust/power"
  [I] -> Mux25/9  "throttle"
  [F] -> Mux25/6  "AHRS"
  [H] -> Mux25/8  "geodesy (all planes)"
  [N] -> Mux25/14  "L/D ratio"
  [P] -> Mux25/16  "cyclics (rotorcraft)"
  [R] -> Mux25/18  "lift/drag"
  [Q] -> Mux25/17  "ground effects"
  [S] -> Mux25/19  "NAVAIDs"
  [T] -> Mux25/20  "switches"
  [V] -> Mux25/22  "autopilot modes"
  [W] -> Mux25/23  "operation systems"
  [Y] -> Mux25/25  "climb/cruise stats"
  [X] -> Terminator/1  "camera/ground values"
  Ground/1 -> Mux25/24
  Ground1/1 -> Mux25/21
  [U] -> Terminator1/1  "annunciators"
  [O] -> Mux25/15  "control deflections"
  Package data string/2(y2) -> Byte Pack/2
  Constant8/1 -> [time]
  Constant10/1 -> [speed]
  Constant1/1 -> [atmos]
  Constant3/1 -> [controls]
  Constant4/1 -> [gear]
  Constant11/1 -> [controls2]
  [controls2] -> Switch13/2, Switch8/2
  Constant15/1 -> [AHRS]
  Constant16/1 -> [geodesy]
  Constant19/1 -> [geodesy2]
  Constant20/1 -> [throttle]
  Constant23/1 -> [eng]
  Constant26/1 -> [prop_sys]
  Constant27/1 -> [weight]
  Constant28/1 -> [forces]
  Constant31/1 -> [cyclics]
  Constant32/1 -> [grnd]
  Constant36/1 -> [NAVAID]
  Constant38/1 -> [autopilots]
  Constant40/1 -> [switches], [op_sys]
  Constant41/1 -> [climb_cruise]
  [op_sys] -> Switch128/2, Switch127/2, Switch126/2, Switch125/2, Switch124/2, Switch123/2, Switch122/2, Switch121/2, Switch120/2, Switch119/2
  Camera/1 -> Switch131/2, Switch130/2, Switch129/2
  Byte Pack/1 -> UDP Send/1
  Package data string/1(y1) -> Byte Pack/1
  Unselect frame rate <0>/2(y2) -> Byte Pack1/2
  Byte Pack1/1 -> UDP Send1/1
  Unselect frame rate <0>/1(y1) -> Byte Pack1/1
  [cyclics] -> Switch79/2, Switch84/2, Switch81/2, Switch80/2
  Constant37/1 -> Switch37/2
  [eng] -> Switch69/2
  [gear] -> Switch64/2
  Constant46/1 -> Switch11/2

== system FlightDataRecorder/Receive X-Plane Data/Speeds ==
  Data : Inport
  Bus Creator : BusCreator  Inputs=6
  Bus Creator1 : BusCreator  Inputs=3
  Demux : Demux  Outputs=8
  Demux1 : Demux  Outputs=8
  Select rows : dspindex/Multiport Selector  rowsOrCols=Rows  idxCellArray={4,5}  idxErrMode=Clip Index
  Terminator{,1..6} (7 alike) : Terminator
  Speeds : Outport
  G-loading : Outport  Port=2
  wires:
  Demux/8 -> Terminator6/1  "Vg (mph)"
  Data/1 -> Select rows/1
  Demux1/8 -> Terminator2/1  "-999"
  Demux/7 -> Terminator5/1  "Vtrue (mph)"
  Bus Creator/1 -> Speeds/1  "Speeds"
  Bus Creator1/1 -> G-loading/1  "G-loading"
  Demux1/4 -> Terminator1/1  "-999"
  Demux1/2 -> Terminator3/1  "-999"
  Demux/6 -> Terminator4/1  "Vind (mph)"
  Select rows/2 -> Demux1/1
  Select rows/1 -> Demux/1
  Demux/5 -> Terminator/1  "-999"
  Demux/1 -> Bus Creator/1  "kias"
  Demux/2 -> Bus Creator/2  "keas"
  Demux/3 -> Bus Creator/3  "ktas"
  Demux/4 -> Bus Creator/4  "ktgs"
  Demux1/1 -> Bus Creator/5  "mach"
  Demux1/3 -> Bus Creator/6  "vvi (fpm)"
  Demux1/6 -> Bus Creator1/1  "gx"
  Demux1/7 -> Bus Creator1/2  "gy"
  Demux1/5 -> Bus Creator1/3  "gz"
